simulink model "phase"  (R2020a)
settings: Solver=VariableStepAuto  StartTime=0.0  StopTime=0.001  RelTol=1e-3
undefined symbols (not defined in the file or in its folder): NBits
libraries: simulink x1, dsparch4 x1, msbAdcArchitectures x1
settings Model: Creator=verty  LastModifiedBy=verty

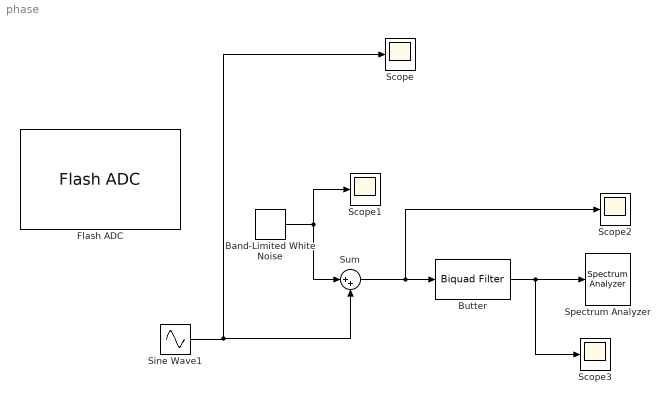
== system phase ==
  Band-Limited White Noise : simulink/Sources/Band-Limited White Noise  Cov=[0.00000001]  Ts=0.000000001  seed=[23341]
  Butter : dsparch4/Biquad Filter  Tag=BlockMethodSubSystem  FilterSource=Dialog parameters  CoeffSource=Specify via dialog  FilterObject=BQF  IIRFiltStruct=Direct form II  BiQuadCoeffs=[0.310774667338081567 0.621549334676163134 0.310774667338081567 1 0.581370401716526874 0.162740803433054249;0.766554848730479743 1.53310969746095949 0.766554848730479743 1 0.855466259447791089 0.710932518895582954;0.52620737654731542 1.05241475309463084 0.52620737654731542 1 0.540720302716684698 0.0814406054333698809;0.78827786268008837 1.57655572536017674 0.78827786268008837 1 0.675156564498150091 0.350313128996300738]  ScaleValues=[0.58137040488115399;1;1;1;1]  IC=0  ICnum=0  ICden=0  a0Flag=Warning  optimizeScaleValues=on  ScaleValueMode=Specify via input port (g)  InputProcessing=Columns as channels (frame based)  roundingMode=Floor  overflowMode=off  scaleValueFracLength=14  denProdOutputFracLength=30  denAccumFracLength=30  secondMemoryFracLength=15
  Flash ADC : msbAdcArchitectures/Flash ADC  NBits=10  InputRange=[-1 1]  ExtStartClk=on  StartFreq=1e6  StartClkJitter=1e-12  Trigger=Rising edge  MatchScale=off  OutputPolarity=Auto  OutDataType=fixdt(1,NBits)  EnableImp=off  OffsetError=3  OffsetErrorUnit=LSB  GainError=2  GainErrorUnit=LSB  Bubbles=[]
      settings: SourceProductBaseCode=AM
  Scope{,1..3} (4 alike) : Scope
  Sine Wave1 : Sin  Amplitude=10  Frequency=2000000  SampleTime=0.0000000001  VectorParams1D=off
  Spectrum Analyzer : SpectrumAnalyzer
  Sum : Sum  Inputs=|++
  wires:
  Band-Limited White Noise/1 -> Scope1/1, Sum/1
  Sum/1 -> Scope2/1, Butter/1
  Butter/1 -> Scope3/1, Spectrum Analyzer/1
  Sine Wave1/1 -> Sum/2, Scope/1
